simulink model "Blink_MultiRate"  (R2018a)
settings: Solver=FixedStepAuto  StartTime=0.0  StopTime=inf  FixedStep=.01  RelTol=1e-3  EnableMultiTasking=on
libraries: arduinolib x3
settings Model: ExtModeTrigDuration=2  Creator=jonathancoulter  LastModifiedBy=jonathancoulter
settings SolverCC: AutoInsertRateTranBlk=on
settings OptimizationCC: DefaultParameterBehavior=Inlined  UseFloatMulNetSlope=on  InlineInvariantSignals=on  PassReuseOutputArgsThreshold=0  EfficientFloat2IntCast=on  MaxStackSize=64
settings DebuggingCC: ParameterTunabilityLossMsg=error
settings HardwareCC: ProdBitPerInt=16  ProdBitPerPointer=16  ProdBitPerSizeT=16  ProdBitPerPtrDiffT=16  ProdLargestAtomicFloat=None  ProdWordSize=8  ProdHWDeviceType=Atmel->AVR  UseEmbeddedCoderFeatures=off
settings SFSimCC: MATLABDynamicMemAlloc=off
settings RTWCC: SystemTargetFile=ert.tlc  HardwareBoard=Arduino Uno  TLCOptions=-aInlineSetEventsForThisBaseRateFcn=TLC_FALSE -aSuppressMultiTaskScheduler=TLC_FALSE -aRateBasedStepFcn=1  TemplateMakefile=ert_default_tmf  Toolchain=Arduino AVR  BuildConfiguration=Faster Runs  CheckMdlBeforeBuild=Warning
settings CodeAppCC: ForceParamTrailComments=on  OperatorAnnotations=on  StateflowObjectComments=on  MATLABSourceComments=on
settings ERTTargetCC: ERTCustomFileBanners=off  SupportNonFinite=off  SupportContinuousTime=on  SupportNonInlinedSFcns=on  RemoveResetFunc=off  SupportVariableSizeSignals=on  ModelStepFunctionPrototypeControlCompliant=off  InlinedParameterPlacement=NonHierarchical

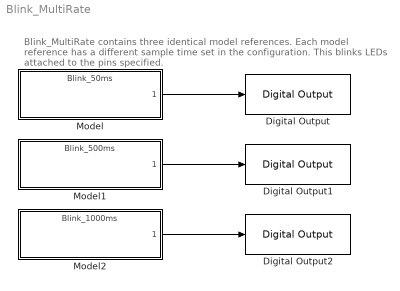
== system Blink_MultiRate ==
  note: Blink_MultiRate contains three identical model references. Each model reference has a different sample time set in the configuration.
      | This blinks LEDs attached to the pins specified.
  Digital Output : arduinolib/Digital Output  pinNumber=13  blockPlatform=arduino
  Digital Output1 : arduinolib/Digital Output  pinNumber=10  blockPlatform=arduino
  Digital Output2 : arduinolib/Digital Output  pinNumber=9  blockPlatform=arduino
  Model : ModelReference  ModelNameDialog=Blink_50ms.slx  ModelReferenceVersion=1.7
  Model1 : ModelReference  ModelNameDialog=Blink_500ms.slx  ModelReferenceVersion=1.8
  Model2 : ModelReference  ModelNameDialog=Blink_1000ms.slx  ModelReferenceVersion=1.8
  wires:
  Model2/1 -> Digital Output2/1
  Model1/1 -> Digital Output1/1
  Model/1 -> Digital Output/1
